simulink model "s360159_sim"  (R2025a)
settings: Solver=VariableStepAuto  StartTime=0.0  StopTime=t_sim  RelTol=1e-3
undefined symbols (not defined in the file): d1, d2, r, Ts
libraries: cstblocks x2, simulink x1
settings Model: Creator=s360159  LastModifiedBy=s360159

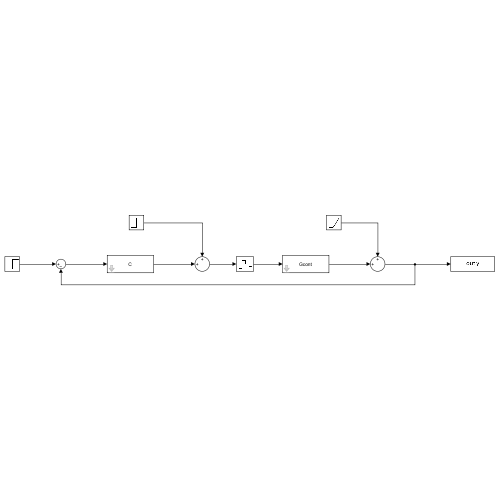
[thumbnail: Simulink's stored preview of the top-level diagram]
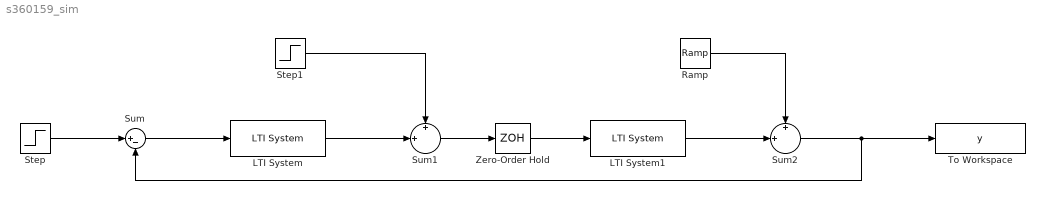
== system s360159_sim ==
  LTI System : cstblocks/LTI System  sys=C  IC=[]  PadeOrder=0
  LTI System1 : cstblocks/LTI System  sys=Gcont  IC=[]  PadeOrder=0
  Ramp : simulink/Sources/Ramp  slope=d2  start=0  InitialOutput=0
  Step : Step  Time=0  After=r  SampleTime=Ts
  Step1 : Step  Time=0  After=d1  SampleTime=Ts
  Sum : Sum  Inputs=|+-
  Sum1 : Sum  Inputs=+|+||
  Sum2 : Sum  Inputs=+|+||
  To Workspace : ToWorkspace  VariableName=y  SaveFormat=Timeseries  SampleTime=Ts
  Zero-Order Hold : ZeroOrderHold  SampleTime=Ts
  wires:
  Step/1 -> Sum/1
  Sum/1 -> LTI System/1
  LTI System/1 -> Sum1/2
  Sum1/1 -> Zero-Order Hold/1
  Zero-Order Hold/1 -> LTI System1/1
  LTI System1/1 -> Sum2/2
  Sum2/1 -> Sum/2, To Workspace/1
  Step1/1 -> Sum1/1
  Ramp/1 -> Sum2/1
